simulink model "LKAS_AutoSave_20200911_1102"  (R2018b)
settings: Solver=FixedStepDiscrete  StartTime=0.0  StopTime=10.0  FixedStep=0.01  RelTol=1e-3
InitFcn:
  | tmpVer = ver('MATLAB');
  | tmpVer = str2num(tmpVer.Version);
  | % -------------------------------------------------------------------
  | %  MATLAB file generated by Simulink.saveVars on 21-Nov-2019 10:06:14
  | %  MATLAB version: 7.13.0.564 (R2011b)
  | % -------------------------------------------------------------------
  | 
  | 
  | SInt16 = Simulink.AliasType;
  | SInt16.Description = 'Num';
  | if (tmpVer > 7.11)
  | 	SInt16.DataScope = 'Auto';
  | end
  | SInt16.HeaderFile = 'Rte_Type.h';
  | SInt16.BaseType = 'int16';
  | 
  | SInt32 = Simulink.AliasType;
  | SInt32.Description = 'Num';
  | if (tmpVer > 7.11)
  | 	SInt32.DataScope = 'Auto';
  | end
  | SInt32.HeaderFile = 'Rte_Type.h';
  | SInt32.BaseType = 'int32';
  | 
  | SInt8 = Simulink.AliasType;
  | SInt8.Description = 'Num';
  | if (tmpVer > 7.11)
  | 	SInt8.DataScope = 'Auto';
  | end
  | SInt8.HeaderFile = 'Rte_Type.h';
  | SInt8.BaseType = 'int8';
  | 
  | T_A_m2_1024_1_u32 = Simulink.NumericType;
  | T_A_m2_1024_1_u32.Description = 'm2 (square meters  (m2))';
  | if (tmpVer > 7.11)
  | 	T_A_m2_1024_1_u32.DataScope = 'Auto';
  | end
  | T_A_m2_1024_1_u32.HeaderFile = 'Rte_Type.h';
  | T_A_m2_1024_1_u32.DataTypeMode = 'Fixed-point: slope and bias scaling';
  | T_A_m2_1024_1_u32.SignednessBool = false;
  | T_A_m2_1024_1_u32.WordLength = 32;
  | T_A_m2_1024_1_u32.FixedExponent = -10;
  | T_A_m2_1024_1_u32.SlopeAdjustmentFactor = 1;
  | T_A_m2_1024_1_u32.Bias = 0;
  | T_A_m2_1024_1_u32.DataTypeOverride = 'Inherit';
  | T_A_m2_1024_1_u32.IsAlias = true;
  | 
  | T_A_m2_65536_1_u16 = Simulink.NumericType;
  | T_A_m2_65536_1_u16.Description = 'm2 (square meters  (m2))';
  | if (tmpVer > 7.11)
  | 	T_A_m2_65536_1_u16.DataScope = 'Auto';
  | end
  | T_A_m2_65536_1_u16.HeaderFile = 'Rte_Type.h';
  | T_A_m2_65536_1_u16.DataTypeMode = 'Fixed-point: slope and bias scaling';
  | T_A_m2_65536_1_u16.SignednessBool = false;
  | T_A_m2_65536_1_u16.WordLength = 16;
  | T_A_m2_65536_1_u16.FixedExponent = -16;
  | T_A_m2_65536_1_u16.SlopeAdjustmentFactor = 1;
  | T_A_m2_65536_1_u16.Bias = 0;
  | T_A_m2_65536_1_u16.DataTypeOverride = 'Inherit';
  | ... (+4598 lines)
StopFcn:
  | clear  T_A_m2_1024_1_u32 T_A_m2_65536_1_u16 T_A_m2_Float32 T_A_mm2_10_1_u16 T_A_mm2_4_1_s16 T_A_mm2_Float32 T_Cnt_Num_10_1_u32 T_Cnt_Num_1_1_s16 T_Cnt_Num_1_1_s32 T_Cnt_Num_1_1_s8 T_Cnt_Num_1_1_u16 T_Cnt_Num_1_1_u32 T_Cnt_Num_1_1_u8 T_E_J_1_1_s32 T_E_J_Float32 T_E_kJ_128_1_s32 T_E_kJ_Float32 T_E_kwh_10_1_u16 T_E_kwh_Float32 T_Epl_kwhpkm_100_1_u16 T_Epl_kwhpkm_Float32 T_F_N_1_1_s16 T_F_N_Float32 T_I_A_1000_1_u16 T_I_A_1048576_1_s32 T_I_A_2048_1_s16 T_I_A_32_1_s16 T_I_A_Float32 T_I_mA_1_1_s16 T_I_mA_32768_128_s16 T_I_mA_Float32 T_J_kgpm2_128_1_u16 T_J_kgpm2_Float32 T_K_NA_1000_1_s16 T_K_NA_100_1_s16 T_K_NA_100_1_u16 T_K_NA_1024_1_s16 T_K_NA_1024_1_u16 T_K_NA_128_1_s16 T_K_NA_128_1_u16 T_K_NA_128_1_u8 T_K_NA_16777216_1_u32 T_K_NA_16_1_s16 T_K_NA_16_1_u16 T_K_NA_16_1_u8 T_K_NA_1_16_u16 T_K_NA_1_1_s16 T_K_NA_1_1_u16 T_K_NA_1_1_u8 T_K_NA_32768_1_s16 T_K_NA_32768_1_u16 T_K_NA_32_1_s8 T_K_NA_4096_1_u16 T_K_NA_4194304_1_s32 T_K_NA_4194304_1_u16 T_K_NA_65536_1_s32 T_K_NA_65536_1_u16 T_K_NA_8192_1_s16 T_K_NA_8_1_s16 T_K_NA_Float32 T_M_Nm_16_1_s16 T_M_Nm_1_1_s16 T_M_Nm_32768_1_s16 T_M_Nm_32_1_s16 T_M_Nm_4_1_s16 T_M_Nm_512_1_s16 T_M_Nm_Float32 T_P_W_1_4_s16 T_P_W_1_8_s16 T_P_W_Float32 T_P_kW_128_1_s16 T_P_kW_1_8_s16 T_P_kW_8_1_s32 T_P_kW_Float32 T_Pct_pct_1024_1_s32 T_Pct_pct_1024_1_u32 T_Pct_pct_10_1_s16 T_Pct_pct_10_1_u32 T_Pct_pct_128_100_s8 T_Pct_pct_1_1_s16 T_Pct_pct_1_4_u8 T_Pct_pct_255_100_u16 T_Pct_pct_255_100_u8 T_Pct_pct_256_1_s16 T_Pct_pct_256_1_u16 T_Pct_pct_65535_100_u16 T_Pct_pct_Float32 T_R_ohm_1024_1_s16 T_R_ohm_32_1_s16 T_R_ohm_Float32 T_TK_K_16_1_s16 T_TK_K_Float32 T_T_degC_10_400_1_u16 T_T_degC_16_1_s16 T_T_degC_1_40_1_u8 T_T_degC_2_80_1_u8 T_T_degC_Float32 T_U_V_1000_1_u16 T_U_V_10_1_u8 T_U_V_200_1_u8 T_U_V_32_1_s16 T_U_V_4096_1_s16 T_U_V_512_1_s16 T_U_V_65535_8_u16 T_U_V_8192_1_u16 T_U_V_Float32 T_U_mV_1_1_s16 T_U_mV_256_20_u16 T_U_mV_Float32 T_V_l_256_1_s16 T_V_l_4096_1_s16 T_V_l_64_1_s16 T_V_l_65535_100_u16 T_V_l_Float32 T_V_ml_128_1_s16 T_V_ml_1_1_s16 T_V_ml_32768_1_s16 T_V_ml_Float32 T_V_ul_32_1_u16 T_V_ul_Float32 T_Vpl_clpkm_512_1_u16 T_Vpl_clpkm_Float32 T_a_kphps_16_1_s16 T_a_kphps_Float32 T_a_mps2_128_1_s16 T_a_mps2_Float32 T_c_MJpkg_256_1_s16 T_c_MJpkg_Float32 T_c_kJpgpK_1024_1_s16 T_c_kJpgpK_Float32 T_c_kJpkgpK_128_1_u16 T_c_kJpkgpK_Float32 T_chrg_Ah_1_1_s16 T_chrg_Ah_1_1_u16 T_chrg_Ah_1_1_u8 T_chrg_Ah_256_1_u16 T_chrg_Ah_4194304_1_s32 T_chrg_Ah_512_1_u16 T_chrg_Ah_8_1_u16 T_chrg_Ah_Float32 T_cmp_NA_100_1_s16 T_cmp_NA_128_1_s16 T_cmp_NA_16_1_s16 T_cmp_NA_32768_1_u16 T_cmp_NA_Float32 T_d2n_rpmps2_4_1_s16 T_d2n_rpmps2_Float32 T_dPct_pctps_16_1_s16 T_dPct_pctps_256_1_s16 T_dPct_pctps_Float32 T_dT_degCps_128_1_s16 T_dT_degCps_Float32 T_dV_lph_1_1_s16 T_dV_lph_Float32 T_dV_lpm_128_1_s16 T_dV_lpm_32_1_s16 T_dV_lpm_Float32 T_dV_lps_1024_1_u16 T_dV_lps_4_1_u16 T_dV_lps_Float32 T_dV_mlps_1024_1_s16 T_dV_mlps_Float32 T_d_BitField16 T_dm_gps_128_1_s16 T_dm_gps_128_1_u16 T_dm_gps_256_1_u16 T_dm_gps_Float32 T_dm_mgps_1_1_s16 T_dm_mgps_Float32 T_dn_rpmps_1_1_s16 T_dn_rpmps_2_1_s16 T_dn_rpmps_Float32 T_dp_Paps_1_1_s16 T_dp_Paps_Float32 T_dp_kPaps_1_1_s16 T_dp_kPaps_8_1_s16 T_dp_kPaps_Float32 T_dphi_degps_128_1_s16 T_dphi_degps_8_1_s16 T_dphi_degps_Float32 T_dr_ps_256_1_s16 T_dr_ps_Float32 T_drho_mgplps_1_2_s16 T_drho_mgplps_Float32 T_e_NA_1_1_u8 T_f_Hz_1_1_u16 T_f_Hz_1_1_u32 T_f_Hz_64_1_u16 T_f_Hz_8_1_s16 T_f_Hz_Float32 T_g_BitField32 T_l_km_16_1_s16 T_l_km_1_1_u16 T_l_km_1_1_u32 T_l_km_Float32 T_l_m_1024_1_s16 T_l_m_16_1_s16 T_l_m_1_1_u32 T_l_m_Float32 T_l_mm_16_1_s16 T_l_mm_1_1_u16 T_l_mm_4096_1_s16 T_l_mm_4_1_u8 T_l_mm_64_1_s16 T_l_mm_Float32 T_m_g_1_1_s16 T_m_g_2048_1_s16 T_m_g_32_1_u16 T_m_g_Float32 T_m_kg_1024_1_s16 T_m_kg_1_1_s16 T_m_kg_1_1_u32 T_m_kg_Float32 T_m_mg_128_1_s16 T_m_mg_32_1_s16 T_m_mg_Float32 T_n_rpm_1_1_s16 T_n_rpm_1_25_u8 T_n_rpm_256_50_u16 T_n_rpm_2_25_u8 T_n_rpm_4_1_u16 T_n_rpm_Float32 T_p_MPa_64_1_s16 T_p_MPa_Float32 T_p_Pa_1_1_s16 T_p_Pa_Float32 T_p_kPa_1_10_u16 T_p_kPa_1_1_s16 T_p_kPa_1_1_u8 T_p_kPa_256_1_u16 T_p_kPa_32_1_u16 T_p_kPa_64_1_s16 T_p_kPa_Float32 T_phi_deg_100_1_s16 T_phi_deg_1024_1_s16 T_phi_deg_128_1_s16 T_phi_deg_1_1_u8 T_phi_deg_256_1_s16 T_phi_deg_2_1_s8 T_phi_deg_32_1_s16 T_phi_deg_512_6_s32 T_phi_deg_Float32 T_phi_rad_2048_1_s16 T_phi_rad_Float32 T_r_NA_1024_1_s16 T_r_NA_1024_1_u16 T_r_NA_16384_1_s16 T_r_NA_16_1_s16 T_r_NA_256_1_s8 T_r_NA_256_1_u16 T_r_NA_32768_1_u16 T_r_NA_32_1_u16 T_r_NA_4096_1_s16 T_r_NA_65535_2_u16 T_r_NA_8192_1_u16 T_r_NA_Float32 T_rho_gpl_8192_1_s16 T_rho_gpl_Float32 T_rho_kgpm3_16_1_s16 T_rho_kgpm3_Float32 T_rho_mgpl_1_1_s16 T_rho_mgpl_64_1_s16 T_rho_mgpl_Float32 T_t_hour_1_1_s16 T_t_hour_Float32 T_t_m_1_1_u16 T_t_m_Float32 T_t_ms_1_1_s16 T_t_ms_1_1_u16 T_t_ms_1_1_u32 T_t_ms_4096_1_s16 T_t_ms_64_1_s16 T_t_ms_Float32 T_t_s_1000_1_s16 T_t_s_100_1_s16 T_t_s_10_1_s16 T_t_s_10_1_u16 T_t_s_1_1_s16 T_t_s_1_1_u16 T_t_s_1_1_u32 T_t_s_Float32 T_t_us_10_1_u32 T_t_us_1_1_s16 T_t_us_1_1_u32 T_t_us_1_4_u16 T_t_us_Float32 T_v_kph_1_1_u8 T_v_kph_64_1_s16 T_v_kph_64_1_u16 T_v_kph_Float32 T_v_mps_256_1_s16 T_v_mps_Float32 T_w_radps_32_1_s16 T_w_radps_Float32 T_y_BitField8 T_y_BitFieldDiagProgress T_y_BitFieldDiagStatus T_y_NA_1_1_u8 SInt16 SInt32 SInt8 T_BOOLEAN UInt16 UInt32 UInt8 s16 s32 s8 u16 u32 u8
model workspace (MAT data in the model file):
  MCOS : class17 (value not decoded)
  MCOS : class17 (value not decoded)
  MCOS : class17 (value not decoded)
  MCOS : class17 (value not decoded)
  MCOS : class17 (value not decoded)
  MCOS : class17 (value not decoded)
  MCOS : class17 (value not decoded)
  MCOS : class17 (value not decoded)
  MCOS : class17 (value not decoded)
  MCOS : class17 (value not decoded)
  MCOS : class17 (value not decoded)
  MCOS : class17 (value not decoded)
  MCOS : class17 (value not decoded)
  MCOS : class17 (value not decoded)
  MCOS : class17 (value not decoded)
  MCOS : class17 (value not decoded)
  MCOS : class17 (value not decoded)
  MCOS : class17 (value not decoded)
  MCOS : class17 (value not decoded)
  MCOS : class17 (value not decoded)
  MCOS : class17 (value not decoded)
  MCOS : class17 (value not decoded)
  MCOS : class17 (value not decoded)
  MCOS : class17 (value not decoded)
  MCOS : class17 (value not decoded)
  MCOS : class17 (value not decoded)
  MCOS : class17 (value not decoded)
  MCOS : class17 (value not decoded)
  MCOS : class17 (value not decoded)
  MCOS : class17 (value not decoded)
  MCOS : class17 (value not decoded)
  MCOS : class17 (value not decoded)
  MCOS : class17 (value not decoded)
  MCOS : class17 (value not decoded)
  MCOS : class17 (value not decoded)
  MCOS : class17 (value not decoded)
  MCOS : class17 (value not decoded)
  MCOS : class17 (value not decoded)
  MCOS : class17 (value not decoded)
  MCOS : class17 (value not decoded)
  MCOS : class17 (value not decoded)
  MCOS : class17 (value not decoded)
  MCOS : class17 (value not decoded)
  MCOS : class17 (value not decoded)
  MCOS : class17 (value not decoded)
  MCOS : class17 (value not decoded)
  MCOS : class17 (value not decoded)
  MCOS : class17 (value not decoded)
  MCOS : class17 (value not decoded)
  MCOS : class17 (value not decoded)
  MCOS : class17 (value not decoded)
  MCOS : class17 (value not decoded)
  MCOS : class17 (value not decoded)
  MCOS : class17 (value not decoded)
  MCOS : class17 (value not decoded)
  MCOS : class17 (value not decoded)
  MCOS : class17 (value not decoded)
  MCOS : class17 (value not decoded)
  MCOS : class17 (value not decoded)
  MCOS : class17 (value not decoded)
  MCOS : class17 (value not decoded)
  MCOS : class17 (value not decoded)
  MCOS : class17 (value not decoded)
  MCOS : class17 (value not decoded)
  MCOS : class17 (value not decoded)
  MCOS : class17 (value not decoded)
  MCOS : class17 (value not decoded)
  MCOS : class17 (value not decoded)
  MCOS : class17 (value not decoded)
  MCOS : class17 (value not decoded)
  MCOS : class17 (value not decoded)
  MCOS : class17 (value not decoded)
  MCOS : class17 (value not decoded)
  MCOS : class17 (value not decoded)
  MCOS : class17 (value not decoded)
  MCOS : class17 (value not decoded)
  MCOS : class17 (value not decoded)
  MCOS : class17 (value not decoded)
  MCOS : class17 (value not decoded)
  MCOS : class17 (value not decoded)
  MCOS : class17 (value not decoded)
  MCOS : class17 (value not decoded)
  MCOS : class17 (value not decoded)
  MCOS : class17 (value not decoded)
  MCOS : class17 (value not decoded)
  MCOS : class17 (value not decoded)
  MCOS : class17 (value not decoded)
  MCOS : class17 (value not decoded)
  MCOS : class17 (value not decoded)
undefined symbols (not defined in the file): LKA_CarWidth, LKA_SampleTime, LKA_StrRatio_C, LKA_Veh2CamL_C, LKA_Veh2CamW_C, LKA_WhlBaseL_C, LL_CompSWA_C, LL_CrvtPrvwT_C, LL_DesDvt_C, LL_DvtComp_C, LL_DvtPrvwT_C, LL_DvtSpdDet_vDvtSpdMin_C, LL_HdAgExT_C, LL_HdAgPrvwT_C, LL_LAccMax_C, LL_LAccRMax_C, LL_LDW_EarliestWarnLine_C, LL_LDW_LatestWarnLine_C, LL_LDWS_SUPPRESS_HEADING, LL_LFClb_TFC_DiffCtlBalance, LL_LFClb_TFC_DiffCtrlMaxSWA, LL_LFClb_TFC_DiffCtrlRatio, LL_LFClb_TFC_facmGainLutGain1_C, LL_LFClb_TFC_facmGainLutGain2_C, LL_LFClb_TFC_facmIntegRatio, LL_LFClb_TFC_facmKlat_C, LL_LFClb_TFC_FfCtlRatio_C, LL_LFClb_TFC_phiIntegCtlMaxSWA_C, LL_LFClb_TFC_tiKlatPrvwT_C, LL_LFClb_TFC_vGainLutVehSpdLwr_C, LL_LFClb_TFC_vGainLutVehSpdUpr_C, LL_LKA_EarliestWarnLine_C, LL_LKA_LatestWarnLine_C, LL_LKAExPrcs_ExitC0Dvt, LL_LKAExPrcs_ExitC0Swt, LL_LKAExPrcs_tiExitTime1, LL_LKAExPrcs_tiExitTime2, LL_LKAExPrcs_tiExitTime3, LL_LKAS_OUT_OF_CONTROL_LAT_VEL, LL_LKAS_OUT_OF_CONTROL_TTLC, LL_LKASWASyn_M0, LL_LKASWASyn_M1, LL_LKASWASyn_M2, LL_LKASWASyn_M3K, LL_LKASWASyn_SWAaddMax, LL_LKASWASyn_T2, LL_LKASWASyn_tiTrqSwaRtTime, LL_LKASWASyn_tiTrqSwaTime, LL_LKASWASyn_TrqMax, LL_LKASWASyn_TrqSwaAddSwt, LL_LKASWASyn_TrqSwaRateDiff, LL_LSpdCompT_C, LL_lStpLngth_C, LL_MAX_DELAY_EPSSTAR_TIME, LL_MAX_DRIVER_TORQUE_DISABLE, LL_MAX_DRIVER_TORQUE_ENABLE, LL_MAX_LANE_WIDTH_DISABLE, LL_MAX_LANE_WIDTH_ENABLE, LL_MAX_LAT_ACC_DISABLE, LL_MAX_LAT_ACC_ENABLE ... (+29)
libraries: simulink x134, dspstat3 x3, simulink_extras x1
(part 11 of 19)

== system LKAS_AutoSave_20200911_1102/LKAS/LL/LLOn/LKA/LKA Exit Processing (LKAExPrcs)/Exit Time 3/Moving Standard Deviation2 ==
  In1 : Inport
  Delay{,1..48} (49 alike) : Delay  DelayLength=1
  Mux : Mux  Inputs=50
  Standard Deviation : dspstat3/Standard Deviation  run=off  directionMode=Entire input  dimension=2  reset_popup=None  roiEnable=off  roiType=Rectangles  roiPortion=Entire ROI  roiOutput=Individual statistics for each ROI  roiFlag=off
      settings: SourceProductName=DSP System Toolbox  SourceProductBaseCode=DS
  Out1 : Outport
  wires:
  In1/1 -> Mux/1, Delay/1
  Delay2/1 -> Mux/4, Delay3/1
  Delay1/1 -> Mux/3, Delay2/1
  Mux/1 -> Standard Deviation/1
  Delay/1 -> Mux/2, Delay1/1
  Standard Deviation/1 -> Out1/1
  Delay3/1 -> Mux/5, Delay4/1
  Delay4/1 -> Mux/6, Delay5/1
  Delay7/1 -> Mux/9, Delay8/1
  Delay6/1 -> Mux/8, Delay7/1
  Delay5/1 -> Mux/7, Delay6/1
  Delay8/1 -> Delay9/1, Mux/10
  Delay18/1 -> Delay28/1, Mux/20
  Delay15/1 -> Mux/17, Delay16/1
  Delay16/1 -> Mux/18, Delay17/1
  Delay17/1 -> Mux/19, Delay18/1
  Delay14/1 -> Mux/16, Delay15/1
  Delay13/1 -> Mux/15, Delay14/1
  Delay10/1 -> Mux/12, Delay11/1
  Delay11/1 -> Mux/13, Delay12/1
  Delay12/1 -> Mux/14, Delay13/1
  Delay9/1 -> Mux/11, Delay10/1
  Delay28/1 -> Mux/21, Delay19/1
  Delay21/1 -> Mux/24, Delay22/1
  Delay20/1 -> Mux/23, Delay21/1
  Delay19/1 -> Mux/22, Delay20/1
  Delay22/1 -> Mux/25, Delay23/1
  Delay23/1 -> Mux/26, Delay24/1
  Delay26/1 -> Mux/29, Delay27/1
  Delay25/1 -> Mux/28, Delay26/1
  Delay24/1 -> Mux/27, Delay25/1
  Delay27/1 -> Delay38/1, Mux/30
  Delay37/1 -> Delay48/1, Mux/40
  Delay34/1 -> Mux/37, Delay35/1
  Delay35/1 -> Mux/38, Delay36/1
  Delay36/1 -> Mux/39, Delay37/1
  Delay33/1 -> Mux/36, Delay34/1
  Delay32/1 -> Mux/35, Delay33/1
  Delay29/1 -> Mux/32, Delay30/1
  Delay30/1 -> Mux/33, Delay31/1
  Delay31/1 -> Mux/34, Delay32/1
  Delay38/1 -> Mux/31, Delay29/1
  Delay48/1 -> Mux/41, Delay39/1
  Delay41/1 -> Mux/44, Delay42/1
  Delay40/1 -> Mux/43, Delay41/1
  Delay39/1 -> Mux/42, Delay40/1
  Delay42/1 -> Mux/45, Delay43/1
  Delay43/1 -> Mux/46, Delay44/1
  Delay46/1 -> Mux/49, Delay47/1
  Delay45/1 -> Mux/48, Delay46/1
  Delay44/1 -> Mux/47, Delay45/1
  Delay47/1 -> Mux/50

== system LKAS_AutoSave_20200911_1102/LKAS/LL/LLOn/LKA/LKA Exit Processing (LKAExPrcs)/Exit Time 3/Sum Condition ==
  In : Inport
  In1 : Inport  Port=2
  Enable : EnablePort  StatesWhenEnabling=reset
  Add1 : Sum  OutDataTypeStr=single
  Data Type Conversion : DataTypeConversion  OutDataTypeStr=uint16
  Memory : Memory  InheritSampleTime=on
  Relational Operator : RelationalOperator  OutDataTypeStr=boolean  RndMeth=Nearest
  Saturation : Saturate  UpperLimit=100000  LowerLimit=0
  Out : Outport  OutputWhenDisabled=reset  InitialOutput=0
  wires:
  Saturation/1 -> Memory/1, Relational Operator/1
  Relational Operator/1 -> Data Type Conversion/1
  Memory/1 -> Add1/2
  Add1/1 -> Saturation/1
  In/1 -> Add1/1
  In1/1 -> Relational Operator/2
  Data Type Conversion/1 -> Out/1

== system LKAS_AutoSave_20200911_1102/LKAS/LL/LLOn/LKA/LKA Exit Processing (LKAExPrcs)/Exit Time 3/Sum Condition1 ==
  In : Inport
  In1 : Inport  Port=2
  Enable : EnablePort  StatesWhenEnabling=reset
  Add1 : Sum  OutDataTypeStr=single
  Data Type Conversion : DataTypeConversion  OutDataTypeStr=uint16
  Memory : Memory  InheritSampleTime=on
  Relational Operator : RelationalOperator  OutDataTypeStr=boolean  RndMeth=Nearest
  Saturation : Saturate  UpperLimit=100000  LowerLimit=0
  Out : Outport  OutputWhenDisabled=reset  InitialOutput=0
  wires:
  Data Type Conversion/1 -> Out/1
  In1/1 -> Relational Operator/2
  In/1 -> Add1/1
  Add1/1 -> Saturation/1
  Memory/1 -> Add1/2
  Relational Operator/1 -> Data Type Conversion/1
  Saturation/1 -> Relational Operator/1, Memory/1

== system LKAS_AutoSave_20200911_1102/LKAS/LL/LLOn/LKA/LKA Motion Planning (LKAMP) /LKA Motion Planning Calculation (LKAMPCal)/Time Division (TDiv) ==
  TDiv_bsTDivInfoOut : Inport
  Add : Sum  OutDataTypeStr=uint16
  Constant : Constant  OutDataTypeStr=uint16  SampleTime=-1
  Constant19 : Constant  OutDataTypeStr=uint16  SampleTime=-1
  If : If  NumInputs=2  IfExpression=u1==u2
  Memory : Memory  InheritSampleTime=on
  Merge : Merge
  Saturation1 : Saturate  UpperLimit=100  LowerLimit=0  OutDataTypeStr=uint16
  if action 1 : Subsystem  TreatAsAtomicUnit=on
  if action 2 : Subsystem  TreatAsAtomicUnit=on
  Out1 : Outport
  wires:
  TDiv_bsTDivInfoOut/1 -> if action 1/1(In1)
  if action 1/1(Out1) -> Merge/2
  Merge/1 -> Out1/1
  if action 2/1(Out1) -> Merge/1
  If/1 -> if action 2/Action
  If/2 -> if action 1/Action
  Memory/1 -> Add/2
  Constant/1 -> Add/1
  Constant19/1 -> If/2
  Add/1 -> Memory/1, Saturation1/1
  Saturation1/1 -> If/1

== system LKAS_AutoSave_20200911_1102/LKAS/LL/LLOn/LKA/LKA Motion Planning (LKAMP) /LKA Motion Planning Calculation (LKAMPCal)/Time Division (TDiv)1 ==
  TDiv_bsTDivInfoOut1 : Inport
  Add : Sum  OutDataTypeStr=uint16
  Constant : Constant  OutDataTypeStr=uint16  SampleTime=-1
  Constant19 : Constant  OutDataTypeStr=uint16  SampleTime=-1
  If : If  NumInputs=2  IfExpression=u1==u2
  Memory : Memory  InheritSampleTime=on
  Merge1 : Merge
  Saturation1 : Saturate  UpperLimit=100  LowerLimit=0  OutDataTypeStr=uint16
  if action 3 : Subsystem  TreatAsAtomicUnit=on
  if action 4 : Subsystem  TreatAsAtomicUnit=on
  Out2 : Outport
  wires:
  Merge1/1 -> Out2/1
  TDiv_bsTDivInfoOut1/1 -> if action 3/1(In1)
  if action 4/1(Out1) -> Merge1/1
  if action 3/1(Out1) -> Merge1/2
  If/2 -> if action 3/Action
  Saturation1/1 -> If/1
  Add/1 -> Saturation1/1, Memory/1
  Constant19/1 -> If/2
  Constant/1 -> Add/1
  Memory/1 -> Add/2
  If/1 -> if action 4/Action

== system LKAS_AutoSave_20200911_1102/LKAS/LL/LLOn/LKA/LKA Motion Planning (LKAMP) /LKA Motion Planning Calculation (LKAMPCal)/Time Division (TDiv)2 ==
  TDiv_bsTDivInfoOut1 : Inport
  Add : Sum  OutDataTypeStr=uint16
  Constant : Constant  OutDataTypeStr=uint16  SampleTime=-1
  Constant19 : Constant  OutDataTypeStr=uint16  SampleTime=-1
  If : If  NumInputs=2  IfExpression=u1==u2
  Memory : Memory  InheritSampleTime=on
  Merge1 : Merge
  Saturation1 : Saturate  UpperLimit=100  LowerLimit=0  OutDataTypeStr=uint16
  if action 3 : Subsystem  TreatAsAtomicUnit=on
  if action 4 : Subsystem  TreatAsAtomicUnit=on
  Out2 : Outport
  wires:
  If/1 -> if action 4/Action
  Memory/1 -> Add/2
  Constant/1 -> Add/1
  Constant19/1 -> If/2
  Add/1 -> Memory/1, Saturation1/1
  Saturation1/1 -> If/1
  If/2 -> if action 3/Action
  if action 3/1(Out1) -> Merge1/2
  if action 4/1(Out1) -> Merge1/1
  TDiv_bsTDivInfoOut1/1 -> if action 3/1(In1)
  Merge1/1 -> Out2/1

== system LKAS_AutoSave_20200911_1102/LKAS/LL/LLOn/LKA/LKA Motion Planning (LKAMP) /LKA Motion Planning Calculation (LKAMPCal)/Time Division (TDiv)3 ==
  TDiv_bsTDivInfoOut1 : Inport
  Add : Sum  OutDataTypeStr=uint16
  Constant : Constant  OutDataTypeStr=uint16  SampleTime=-1
  Constant19 : Constant  OutDataTypeStr=uint16  SampleTime=-1
  If : If  NumInputs=2  IfExpression=u1==u2
  Memory : Memory  InheritSampleTime=on
  Merge1 : Merge
  Saturation1 : Saturate  UpperLimit=100  LowerLimit=0  OutDataTypeStr=uint16
  if action 3 : Subsystem  TreatAsAtomicUnit=on
  if action 4 : Subsystem  TreatAsAtomicUnit=on
  Out2 : Outport
  wires:
  Merge1/1 -> Out2/1
  TDiv_bsTDivInfoOut1/1 -> if action 3/1(In1)
  if action 4/1(Out1) -> Merge1/1
  if action 3/1(Out1) -> Merge1/2
  If/2 -> if action 3/Action
  Saturation1/1 -> If/1
  Add/1 -> Saturation1/1, Memory/1
  Constant19/1 -> If/2
  Constant/1 -> Add/1
  Memory/1 -> Add/2
  If/1 -> if action 4/Action

== system LKAS_AutoSave_20200911_1102/LKAS/LL/LLOn/LKA/LKA Motion Planning (LKAMP) /LKA Motion Planning Calculation (LKAMPCal)/Time Division (TDiv)4 ==
  TDiv_bsTDivInfoOut1 : Inport
  Add : Sum  OutDataTypeStr=uint16
  Constant : Constant  OutDataTypeStr=uint16  SampleTime=-1
  Constant19 : Constant  OutDataTypeStr=uint16  SampleTime=-1
  If : If  NumInputs=2  IfExpression=u1==u2
  Memory : Memory  InheritSampleTime=on
  Merge1 : Merge
  Saturation1 : Saturate  UpperLimit=100  LowerLimit=0  OutDataTypeStr=uint16
  if action 3 : Subsystem  TreatAsAtomicUnit=on
  if action 4 : Subsystem  TreatAsAtomicUnit=on
  Out2 : Outport
  wires:
  If/1 -> if action 4/Action
  Memory/1 -> Add/2
  Constant/1 -> Add/1
  Constant19/1 -> If/2
  Add/1 -> Memory/1, Saturation1/1
  Saturation1/1 -> If/1
  If/2 -> if action 3/Action
  if action 3/1(Out1) -> Merge1/2
  if action 4/1(Out1) -> Merge1/1
  TDiv_bsTDivInfoOut1/1 -> if action 3/1(In1)
  Merge1/1 -> Out2/1

== system LKAS_AutoSave_20200911_1102/LKAS/LL/LLOn/LKA/LKA Motion Planning (LKAMP) /Motion Planning Input Processing (MPInP)/Lane Information Selection (LaneInfoSel) ==
  LaneInfoSel_stLKAActvFlg : Inport
  LaneInfoSel_facmLftLane : Inport  Port=2
  LaneInfoSel_facmRgtLane : Inport  Port=3
  If : If  IfExpression=u1==1  ElseIfExpressions=u1==2
  If Action Subsystem1 : Subsystem  TreatAsAtomicUnit=on
  If Action Subsystem2 : Subsystem  TreatAsAtomicUnit=on
  If Action Subsystem3 : Subsystem  TreatAsAtomicUnit=on
  Merge : Merge  Inputs=3
  LaneInfoSel_facmActvLane : Outport
  wires:
  LaneInfoSel_facmRgtLane/1 -> If Action Subsystem1/1(In1)
  LaneInfoSel_facmLftLane/1 -> If Action Subsystem2/1(In1)
  LaneInfoSel_stLKAActvFlg/1 -> If/1
  If/1 -> If Action Subsystem2/Action
  If Action Subsystem2/1(Out1) -> Merge/1
  Merge/1 -> LaneInfoSel_facmActvLane/1
  If/2 -> If Action Subsystem1/Action
  If Action Subsystem1/1(Out1) -> Merge/2
  If Action Subsystem3/1(Out1) -> Merge/3
  If/3 -> If Action Subsystem3/Action

== system LKAS_AutoSave_20200911_1102/LKAS/LL/LLOn/LKA/LKA Motion Planning (LKAMP) /Motion Planning Input Processing (MPInP)/Signal Latching2 ==
  In : Inport
  Add : Sum  OutDataTypeStr=uint16
  Constant : Constant  OutDataTypeStr=uint16  SampleTime=-1
  Constant2 : Constant  Value=LatchTime  OutDataTypeStr=uint16  SampleTime=-1
  If : If  NumInputs=2  IfExpression=u1==u2  ShowElse=off
  Memory : Memory  InheritSampleTime=on
  Saturation1 : Saturate  UpperLimit=10000  LowerLimit=0  OutDataTypeStr=uint16
  "if action " : Subsystem  TreatAsAtomicUnit=on
  Out : Outport
  wires:
  Constant2/1 -> If/2
  In/1 -> "if action "/1(In)
  "if action "/1(Out) -> Out/1
  If/1 -> "if action "/Action
  Constant/1 -> Add/1
  Add/1 -> Saturation1/1
  Memory/1 -> Add/2
  Saturation1/1 -> Memory/1, If/1

== system LKAS_AutoSave_20200911_1102/LKAS/LL/LLOn/LKA/LKA Motion Planning (LKAMP) /Motion Planning Input Processing (MPInP)/Signal Latching3 ==
  In : Inport
  Add : Sum  OutDataTypeStr=uint16
  Constant : Constant  OutDataTypeStr=uint16  SampleTime=-1
  Constant2 : Constant  Value=LatchTime  OutDataTypeStr=uint16  SampleTime=-1
  If : If  NumInputs=2  IfExpression=u1==u2  ShowElse=off
  Memory : Memory  InheritSampleTime=on
  Saturation1 : Saturate  UpperLimit=10000  LowerLimit=0  OutDataTypeStr=uint16
  "if action " : Subsystem  TreatAsAtomicUnit=on
  Out : Outport
  wires:
  Saturation1/1 -> If/1, Memory/1
  Memory/1 -> Add/2
  Add/1 -> Saturation1/1
  Constant/1 -> Add/1
  If/1 -> "if action "/Action
  "if action "/1(Out) -> Out/1
  In/1 -> "if action "/1(In)
  Constant2/1 -> If/2

== system LKAS_AutoSave_20200911_1102/LKAS/LL/LLOn/LKA/LKA Motion Planning (LKAMP) /Motion Planning Input Processing (MPInP)/Signal Latching4 ==
  In : Inport
  Add : Sum  OutDataTypeStr=uint16
  Constant : Constant  OutDataTypeStr=uint16  SampleTime=-1
  Constant2 : Constant  Value=LatchTime  OutDataTypeStr=uint16  SampleTime=-1
  If : If  NumInputs=2  IfExpression=u1==u2  ShowElse=off
  Memory : Memory  InheritSampleTime=on
  Saturation1 : Saturate  UpperLimit=10000  LowerLimit=0  OutDataTypeStr=uint16
  "if action " : Subsystem  TreatAsAtomicUnit=on
  Out : Outport
  wires:
  Constant2/1 -> If/2
  In/1 -> "if action "/1(In)
  "if action "/1(Out) -> Out/1
  If/1 -> "if action "/Action
  Constant/1 -> Add/1
  Add/1 -> Saturation1/1
  Memory/1 -> Add/2
  Saturation1/1 -> Memory/1, If/1

== system LKAS_AutoSave_20200911_1102/LKAS/LL/LLOn/LKA/LKA Motion Planning (LKAMP) /Motion Planning Input Processing (MPInP)/Signal Latching5 ==
  In : Inport
  Add : Sum  OutDataTypeStr=uint16
  Constant : Constant  OutDataTypeStr=uint16  SampleTime=-1
  Constant2 : Constant  Value=LatchTime  OutDataTypeStr=uint16  SampleTime=-1
  If : If  NumInputs=2  IfExpression=u1==u2  ShowElse=off
  Memory : Memory  InheritSampleTime=on
  Saturation1 : Saturate  UpperLimit=10000  LowerLimit=0  OutDataTypeStr=uint16
  "if action " : Subsystem  TreatAsAtomicUnit=on
  Out : Outport
  wires:
  Constant2/1 -> If/2
  In/1 -> "if action "/1(In)
  "if action "/1(Out) -> Out/1
  If/1 -> "if action "/Action
  Constant/1 -> Add/1
  Add/1 -> Saturation1/1
  Memory/1 -> Add/2
  Saturation1/1 -> Memory/1, If/1

== system LKAS_AutoSave_20200911_1102/LKAS/LL/LLOn/LKA/LKA Motion Planning (LKAMP) /Motion Planning Input Processing (MPInP)/Signal Latching6 ==
  In : Inport
  Add : Sum  OutDataTypeStr=uint16
  Constant : Constant  OutDataTypeStr=uint16  SampleTime=-1
  Constant2 : Constant  Value=LatchTime  OutDataTypeStr=uint16  SampleTime=-1
  If : If  NumInputs=2  IfExpression=u1==u2  ShowElse=off
  Memory : Memory  InheritSampleTime=on
  Saturation1 : Saturate  UpperLimit=10000  LowerLimit=0  OutDataTypeStr=uint16
  "if action " : Subsystem  TreatAsAtomicUnit=on
  Out : Outport
  wires:
  Constant2/1 -> If/2
  In/1 -> "if action "/1(In)
  "if action "/1(Out) -> Out/1
  If/1 -> "if action "/Action
  Constant/1 -> Add/1
  Add/1 -> Saturation1/1
  Memory/1 -> Add/2
  Saturation1/1 -> Memory/1, If/1

== system LKAS_AutoSave_20200911_1102/LKAS/LL/LLOn/LKA/LKA Motion Planning (LKAMP) /Motion Planning Input Processing (MPInP)/Signal Latching7 ==
  In : Inport
  Add : Sum  OutDataTypeStr=uint16
  Constant : Constant  OutDataTypeStr=uint16  SampleTime=-1
  Constant2 : Constant  Value=LatchTime  OutDataTypeStr=uint16  SampleTime=-1
  If : If  NumInputs=2  IfExpression=u1==u2  ShowElse=off
  Memory : Memory  InheritSampleTime=on
  Saturation1 : Saturate  UpperLimit=10000  LowerLimit=0  OutDataTypeStr=uint16
  "if action " : Subsystem  TreatAsAtomicUnit=on
  Out : Outport
  wires:
  Saturation1/1 -> If/1, Memory/1
  Memory/1 -> Add/2
  Add/1 -> Saturation1/1
  Constant/1 -> Add/1
  If/1 -> "if action "/Action
  "if action "/1(Out) -> Out/1
  In/1 -> "if action "/1(In)
  Constant2/1 -> If/2

== system LKAS_AutoSave_20200911_1102/LKAS/LL/LLOn/LKA/LKA Motion Planning (LKAMP) /Motion Planning Input Processing (MPInP)/Subsystem ==
  In1 : Inport
  If : If  IfExpression=u1==1  ElseIfExpressions=u1==2
  If Action Subsystem1 : Subsystem  TreatAsAtomicUnit=on
  If Action Subsystem2 : Subsystem  TreatAsAtomicUnit=on
  If Action Subsystem3 : Subsystem  TreatAsAtomicUnit=on
  Merge : Merge  Inputs=3
  Out6 : Outport
  wires:
  If/3 -> If Action Subsystem3/Action
  If Action Subsystem3/1(Out1) -> Merge/3
  If Action Subsystem1/1(Out1) -> Merge/2
  If/2 -> If Action Subsystem1/Action
  Merge/1 -> Out6/1
  If Action Subsystem2/1(Out1) -> Merge/1
  If/1 -> If Action Subsystem2/Action
  In1/1 -> If/1

== system LKAS_AutoSave_20200911_1102/LKAS/LL/LLOn/LKA/LKA Motion Planning (LKAMP) /Switching Condition (SwtCon)/Ending Heading Angle Determination (EndHdAgDet) ==
  EndHdAgDet_stLKAActvFlg : Inport
  EndHdAgDet_vVehSpd : Inport  Port=2
  EndHdAgDet_crPrvwCrvt : Inport  Port=3
  EndHdAgDet_lLaneWidth_C : Inport  Port=4
  EndHdAgDet_lCarWidth_C : Inport  Port=5
  EndHdAgDet_tiHdAgExTime_C : Inport  Port=6
  EndHdAgDet_tiLSpdCompT_C : Inport  Port=7
  Add : Sum  Inputs=+-  OutDataTypeStr=single
  Add1 : Sum  OutDataTypeStr=single
  Divide : Product  Inputs=/*  OutDataTypeStr=single
  Divide1 : Product  Inputs=*/  OutDataTypeStr=single
  Lateral Speed Compensation (LSpdComp) : Subsystem
  kph To mps : Gain  Gain=1/3.6  OutDataTypeStr=single
  EndHdAgDet_phiHdAgMax : Outport
  wires:
  EndHdAgDet_tiLSpdCompT_C/1 -> Lateral Speed Compensation (LSpdComp)/4(LSpdComp_tiLSpdCompT_C)
  EndHdAgDet_crPrvwCrvt/1 -> Lateral Speed Compensation (LSpdComp)/3(LSpdComp_crPrvwCrvt)
  Add1/1 -> EndHdAgDet_phiHdAgMax/1
  Divide1/1 -> Add1/1
  Lateral Speed Compensation (LSpdComp)/1(LSpdComp_phiLSpdComp) -> Add1/2
  Add/1 -> Divide/2
  EndHdAgDet_stLKAActvFlg/1 -> Lateral Speed Compensation (LSpdComp)/2(LSpdComp_stLKAFlg)
  EndHdAgDet_vVehSpd/1 -> kph To mps/1
  EndHdAgDet_tiHdAgExTime_C/1 -> Divide/1
  kph To mps/1 -> Divide1/2, Lateral Speed Compensation (LSpdComp)/1(LSpdComp_vVehSpd)
  EndHdAgDet_lCarWidth_C/1 -> Add/2
  EndHdAgDet_lLaneWidth_C/1 -> Add/1
  Divide/1 -> Divide1/1

== system LKAS_AutoSave_20200911_1102/LKAS/LL/LLOn/LKA/LKA Motion Planning (LKAMP) /Switching Condition (SwtCon)/If Action Subsystem ==
  In1 : Inport
  Action Port : ActionPort  InitializeStates=reset  ActionType=then
  Gain2 : Gain  Gain=-1  OutDataTypeStr=Inherit: Same as input
  Out1 : Outport
  wires:
  In1/1 -> Gain2/1
  Gain2/1 -> Out1/1  "HdAgMax"

== system LKAS_AutoSave_20200911_1102/LKAS/LL/LLOn/LKA/LKA Motion Planning (LKAMP) /Switching Condition (SwtCon)/If Action Subsystem1 ==
  In1 : Inport
  Action Port : ActionPort  InitializeStates=reset  ActionType=elseif
  Cast To Single1 : DataTypeConversion  LockScale=on
  Out1 : Outport
  wires:
  In1/1 -> Cast To Single1/1
  Cast To Single1/1 -> Out1/1  "HdAgMax"

== system LKAS_AutoSave_20200911_1102/LKAS/LL/LLOn/LKA/LKA Motion Planning (LKAMP) /Switching Condition (SwtCon)/If Action Subsystem2 ==
  Action Port : ActionPort  InitializeStates=reset  ActionType=else
  Constant2 : Constant  Value=0  OutDataTypeStr=single  SampleTime=-1
  Out1 : Outport
  wires:
  Constant2/1 -> Out1/1  "HdAgMax"

== system LKAS_AutoSave_20200911_1102/LKAS/LL/LLOn/LKA/LKA Motion Planning (LKAMP) /Switching Condition (SwtCon)/Signal Latching ==
  In : Inport
  Add : Sum  OutDataTypeStr=uint16
  Constant : Constant  OutDataTypeStr=uint16  SampleTime=-1
  Constant2 : Constant  Value=LatchTime  OutDataTypeStr=uint16  SampleTime=-1
  If : If  NumInputs=2  IfExpression=u1==u2  ShowElse=off
  Memory : Memory  InheritSampleTime=on
  Saturation1 : Saturate  UpperLimit=10000  LowerLimit=0  OutDataTypeStr=uint16
  "if action " : Subsystem  TreatAsAtomicUnit=on
  Out : Outport
  wires:
  Constant2/1 -> If/2
  In/1 -> "if action "/1(In)
  "if action "/1(Out) -> Out/1
  If/1 -> "if action "/Action
  Constant/1 -> Add/1
  Add/1 -> Memory/1, Saturation1/1
  Memory/1 -> Add/2
  Saturation1/1 -> If/1

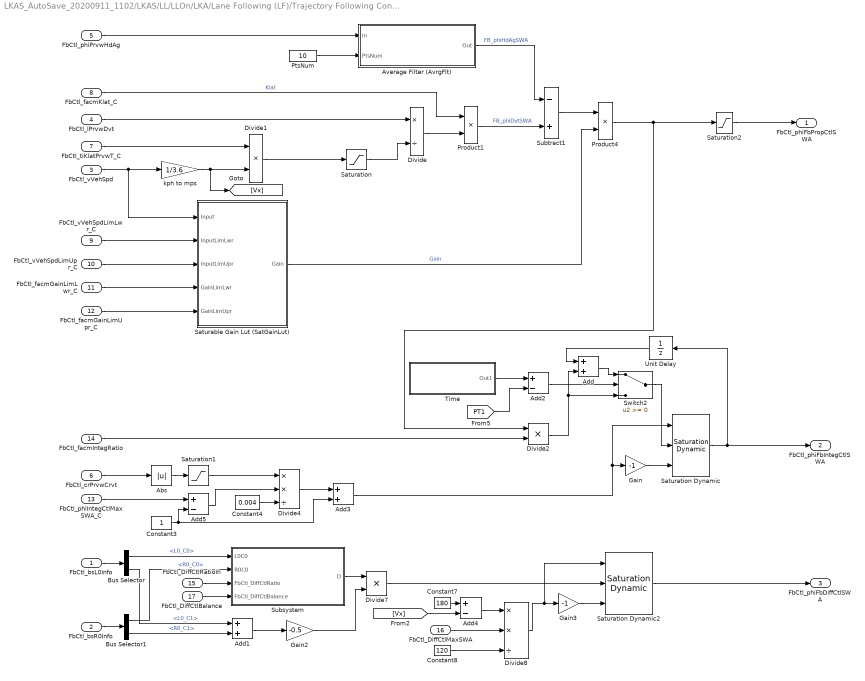
== system LKAS_AutoSave_20200911_1102/LKAS/LL/LLOn/LKA/Lane Following (LF)/Trajectory Following Control (TFC)/Feedback Control (FbCtl) ==
  FbCtl_bsL0Info : Inport
  FbCtl_bsR0Info : Inport  Port=2
  FbCtl_vVehSpd : Inport  Port=3
  FbCtl_lPrvwDvt : Inport  Port=4
  FbCtl_phiPrvwHdAg : Inport  Port=5
  FbCtl_crPrvwCrvt : Inport  Port=6
  FbCtl_tiKlatPrvwT_C : Inport  Port=7
  FbCtl_facmKlat_C : Inport  Port=8
  FbCtl_vVehSpdLimLwr_C : Inport  Port=9
  FbCtl_vVehSpdLimUpr_C : Inport  Port=10
  FbCtl_facmGainLimLwr_C : Inport  Port=11
  FbCtl_facmGainLimUpr_C : Inport  Port=12
  FbCtl_phiIntegCtlMaxSWA_C : Inport  Port=13
  FbCtl_facmIntegRatio : Inport  Port=14
  FbCtl_DiffCtlRatioIn : Inport  Port=15
  FbCtl_DiffCtlMaxSWA : Inport  Port=16
  FbCtl_DiffCtlBalance : Inport  Port=17
  Abs : Abs
  Add : Sum
  Add1 : Sum
  Add2 : Sum  Inputs=+-
  Add3 : Sum
  Add4 : Sum  Inputs=+-
  Add5 : Sum  Inputs=+-
  Average Filter (AvrgFlt) : Subsystem
      mask Display:
      | port_label('input', 1, 'In');
      | port_label('input', 2, 'PtsNum');
      | port_label('output', 1, 'Out');
      | color('blue');
      | text(0.98,0.9,'VCDC Block','horizontalAlignment','right');
      | color('black');
      | text(0.5,0.55,'Average Filter','horizontalAlignment','center');
      | text(0.5,0.4,'(AvrgFlt)','horizontalAlignment','center');
  Bus Selector : BusSelector  OutputSignals=L0_C0,L0_C1
  Bus Selector1 : BusSelector  OutputSignals=R0_C0,R0_C1
  Constant3 : Constant  OutDataTypeStr=single
  Constant4 : Constant  Value=0.004  OutDataTypeStr=single
  Constant7 : Constant  Value=180  OutDataTypeStr=single
  Constant8 : Constant  Value=120  OutDataTypeStr=single
  Divide : Product  Inputs=*/
  Divide1 : Product  Inputs=**
  Divide2 : Product  Inputs=**
  Divide4 : Product  Inputs=**/
  Divide7 : Product  Inputs=**
  Divide8 : Product  Inputs=**/
  Gain : Gain  Gain=-1  OutDataTypeStr=single
  Gain2 : Gain  Gain=-0.5
  Gain3 : Gain  Gain=-1  OutDataTypeStr=single
  Product1 : Product  OutDataTypeStr=single  RndMeth=Zero
  Product4 : Product  OutDataTypeStr=single  RndMeth=Zero
  PtsNum : Constant  Value=10  OutDataTypeStr=single
  Saturable Gain Lut (SatGainLut) : MATLAB Function  TreatAsAtomicUnit=on
  Saturation : Saturate  UpperLimit=40  LowerLimit=5
  Saturation Dynamic : simulink/Discontinuities/Saturation Dynamic  OutMin=[]  OutMax=[]  OutDataTypeStr=Inherit: Same as second input  OutDataType=fixdt(1, 16)  OutScaling=2^-10  DoSatur=off
  Saturation Dynamic2 : simulink/Discontinuities/Saturation Dynamic  OutMin=[]  OutMax=[]  OutDataTypeStr=Inherit: Same as second input  OutDataType=fixdt(1, 16)  OutScaling=2^-10  DoSatur=off
  Saturation1 : Saturate  UpperLimit=0.004  LowerLimit=0.00001
  Saturation2 : Saturate  UpperLimit=360  LowerLimit=-360  OutDataTypeStr=single
  Subsystem : Subsystem
  Subtract1 : Sum  Inputs=-+
  Switch2 : Switch
  Time : Subsystem
      mask Display:
      | port_label('output', 1, 'TTime');
      | color('blue');
      | text(0.98,0.9,'VCDC Block','horizontalAlignment','right');
      | color('black');
      | text(0.5,0.55,'Tick Time','horizontalAlignment','center');
      | text(0.5,0.4,'(TTime)','horizontalAlignment','center');
  Unit Delay : UnitDelay  SampleTime=-1
  kph to mps : Gain  Gain=1/3.6  OutDataTypeStr=single
  FbCtl_phiFbPropCtlSWA : Outport
  FbCtl_phiFbIntegCtlSWA : Outport  Port=2
  FbCtl_phiFbDiffCtlSWA : Outport  Port=3
  wires:
  Gain2/1 -> Divide7/2
  Bus Selector1/1 -> Subsystem/2(R0C0)  "<R0_C0>"
  Bus Selector/1 -> Subsystem/1(L0C0)  "<L0_C0>"
  FbCtl_bsR0Info/1 -> Bus Selector1/1
  FbCtl_bsL0Info/1 -> Bus Selector/1
  PtsNum/1 -> Average Filter (AvrgFlt)/2(PtsNum)
  FbCtl_facmKlat_C/1 -> Product1/1  "Klat"
  Product1/1 -> Subtract1/2  "FB_phiDvtSWA"
  Average Filter (AvrgFlt)/1(Out) -> Subtract1/1  "FB_phiHdAgSWA"
  Saturable Gain Lut (SatGainLut)/1(Gain) -> Product4/2  "Gain"
  Saturation2/1 -> FbCtl_phiFbPropCtlSWA/1
  Saturation/1 -> Divide/2
  Divide1/1 -> Saturation/1
  FbCtl_tiKlatPrvwT_C/1 -> Divide1/1
  FbCtl_lPrvwDvt/1 -> Divide/1
  Divide/1 -> Product1/2
  FbCtl_phiPrvwHdAg/1 -> Average Filter (AvrgFlt)/1(In)
  Product4/1 -> Divide2/1, Saturation2/1
  kph to mps/1 -> Divide1/2, [Vx]
  FbCtl_vVehSpdLimLwr_C/1 -> Saturable Gain Lut (SatGainLut)/2(InputLimLwr)
  FbCtl_vVehSpdLimUpr_C/1 -> Saturable Gain Lut (SatGainLut)/3(InputLimUpr)
  FbCtl_facmGainLimLwr_C/1 -> Saturable Gain Lut (SatGainLut)/4(GainLimLwr)
  FbCtl_facmGainLimUpr_C/1 -> Saturable Gain Lut (SatGainLut)/5(GainLimUpr)
  FbCtl_facmIntegRatio/1 -> Divide2/2
  Divide2/1 -> Add/2, Switch2/3
  Subtract1/1 -> Product4/1
  Add3/1 -> Saturation Dynamic/1, Gain/1
  FbCtl_phiIntegCtlMaxSWA_C/1 -> Add5/1
  FbCtl_vVehSpd/1 -> kph to mps/1, Saturable Gain Lut (SatGainLut)/1(Input)
  Unit Delay/1 -> Add/1
  Gain/1 -> Saturation Dynamic/3
  Saturation Dynamic/1 -> FbCtl_phiFbIntegCtlSWA/1, Unit Delay/1
  Divide7/1 -> Saturation Dynamic2/2
  Gain3/1 -> Saturation Dynamic2/3
  Divide8/1 -> Gain3/1, Saturation Dynamic2/1
  FbCtl_DiffCtlMaxSWA/1 -> Divide8/2
  Constant7/1 -> Add4/1
  Add4/1 -> Divide8/1
  Constant8/1 -> Divide8/3
  [Vx] -> Add4/2
  Bus Selector/2 -> Add1/1  "<L0_C1>"
  Add1/1 -> Gain2/1
  Bus Selector1/2 -> Add1/2  "<R0_C1>"
  Subsystem/1(D) -> Divide7/1
  FbCtl_DiffCtlRatioIn/1 -> Subsystem/3(FbCtl_DiffCtlRatio)
  Saturation Dynamic2/1 -> FbCtl_phiFbDiffCtlSWA/1
  Time/1(Out1) -> Add2/1
  [PT1] -> Add2/2
  Add2/1 -> Switch2/2
  Switch2/1 -> Saturation Dynamic/2
  Add/1 -> Switch2/1
  FbCtl_crPrvwCrvt/1 -> Abs/1
  Abs/1 -> Saturation1/1
  Constant3/1 -> Add5/2, Add3/2
  Saturation1/1 -> Divide4/1
  Divide4/1 -> Add3/1
  Constant4/1 -> Divide4/3
  Add5/1 -> Divide4/2
  FbCtl_DiffCtlBalance/1 -> Subsystem/4(FbCtl_DiffCtlBalance)

== system LKAS_AutoSave_20200911_1102/LKAS/LL/LLOn/LKA/Lane Following (LF)/Trajectory Following Control (TFC)/Feedforward Control (FfCtl) ==
  FfCtl_FfCtlRatio_C : Inport
  FfCtl_vVehSpd : Inport  Port=2
  FfCtl_crPrvwCrvt : Inport  Port=3
  FfCtl_lWhlBase_SY : Inport  Port=4
  FfCtl_rTraRatio_C : Inport  Port=5
  Add : Sum  OutDataTypeStr=single
  Constant1 : Constant  OutDataTypeStr=single
  Divide : Product  Inputs=*/  OutDataTypeStr=single
  Divide1 : Product  Inputs=*/  OutDataTypeStr=single
  Gain2 : Gain  Gain=-1  OutDataTypeStr=single
  Lookup Table2 : Lookup_n-D  NumberOfTableDimensions=1  BreakpointsForDimension1=[11.7,18.83,26.98,31.98,51.04,79,86.08,90.59]  BeginIndexSearchUsingPreviousIndexResult=on  Table=[0.012141,0.005179,0.00298,0.002547,0.001715,0.001283,0.001021,0.000982]  DiagnosticForOutOfRangeInput=Warning  RemoveProtectionInput=on  InternalRulePriority=Speed  OutDataTypeStr=single  InputSameDT=on
  Math Function : Math  Operator=magnitude^2  OutDataTypeStr=single  SaturateOnIntegerOverflow=on
  Product : Product  OutDataTypeStr=single
  Product1 : Product  OutDataTypeStr=single
  Product2 : Product  OutDataTypeStr=single
  Product3 : Product  Inputs=3  OutDataTypeStr=single
  Saturation1 : Saturate  UpperLimit=0.01  LowerLimit=0
  kph to mps : Gain  Gain=1/3.6  OutDataTypeStr=single
  rad to deg : Gain  Gain=180/pi  OutDataTypeStr=single
  FfCtl_phiFfSWA : Outport
  wires:
  Gain2/1 -> FfCtl_phiFfSWA/1
  kph to mps/1 -> Divide/1, Math Function/1, Product/1
  rad to deg/1 -> Product1/1
  Product1/1 -> Product3/2
  Divide1/1 -> Product1/2
  Divide/1 -> Divide1/2
  FfCtl_lWhlBase_SY/1 -> Divide/2
  Add/1 -> Divide1/1
  Constant1/1 -> Add/2
  Product2/1 -> Add/1
  Math Function/1 -> Product2/1
  Product/1 -> rad to deg/1
  FfCtl_crPrvwCrvt/1 -> Product/2
  FfCtl_vVehSpd/1 -> Lookup Table2/1, kph to mps/1
  Product3/1 -> Gain2/1
  FfCtl_rTraRatio_C/1 -> Product3/3
  FfCtl_FfCtlRatio_C/1 -> Product3/1
  Lookup Table2/1 -> Saturation1/1
  Saturation1/1 -> Product2/2  "FfCtl_facmUSG_C"

== system LKAS_AutoSave_20200911_1102/LKAS/LL/LLOn/LKA/Plan To LaneFollowing (PTLF)/InsideJudge1/If Action Subsystem ==
  T1 : Inport
  Plan : Inport  Port=2
  HdAgLft : Inport  Port=3
  Time : Inport  Port=4
  Action Port : ActionPort  InitializeStates=reset  ActionType=then
  Add : Sum
  Cast To Single : DataTypeConversion  OutDataTypeStr=uint8
  Compare To Constant : simulink/Logic and Bit Operations/Compare To Constant  relop=>=  const=0  OutDataTypeStr=boolean
  Detect Decrease : simulink/Logic and Bit Operations/Detect Decrease  vinit=0.0  OutDataTypeStr=boolean
  If Action Subsystem : Subsystem  TreatAsAtomicUnit=on
  If Action Subsystem2 : Subsystem  TreatAsAtomicUnit=on
  Logical Operator : Logic  AllPortsSameDT=off  OutDataTypeStr=boolean
  Memory : Memory  InheritSampleTime=on
  Relational Operator : RelationalOperator  OutDataTypeStr=boolean  RndMeth=Simplest
  Saturation : Saturate  UpperLimit=5  LowerLimit=0
  Switch : Switch  Criteria=u2 > Threshold
  Switch1 : Switch  Criteria=u2 > Threshold
  T1_1 : Outport
  Plan_1 : Outport  Port=2
  wires:
  HdAgLft/1 -> Compare To Constant/1
  Compare To Constant/1 -> Detect Decrease/1
  Time/1 -> If Action Subsystem/1(T1), Relational Operator/2
  Plan/1 -> If Action Subsystem2/2(Plan), If Action Subsystem/2(Plan)
  T1/1 -> If Action Subsystem2/1(T1), Relational Operator/1
  Detect Decrease/1 -> Logical Operator/1
  Relational Operator/1 -> Logical Operator/2
  Add/1 -> Saturation/1
  Memory/1 -> Add/2
  Logical Operator/1 -> Cast To Single/1
  Cast To Single/1 -> Add/1
  Saturation/1 -> Switch1/2, Switch/2, If Action Subsystem/Enable, Memory/1
  If Action Subsystem/1(T1_1) -> Switch/1
  If Action Subsystem/2(Plan_1) -> Switch1/1
  If Action Subsystem2/1(T1_1) -> Switch/3
  If Action Subsystem2/2(Plan_1) -> Switch1/3
  Switch/1 -> T1_1/1
  Switch1/1 -> Plan_1/1

== system LKAS_AutoSave_20200911_1102/LKAS/LL/LLOn/LKA/Plan To LaneFollowing (PTLF)/InsideJudge1/If Action Subsystem1 ==
  T1 : Inport
  Plan : Inport  Port=2
  HdAgRgt : Inport  Port=3
  Time : Inport  Port=4
  Action Port : ActionPort  InitializeStates=reset  ActionType=elseif
  Add : Sum
  Cast To Single : DataTypeConversion  OutDataTypeStr=uint8
  Compare To Constant : simulink/Logic and Bit Operations/Compare To Constant  relop=<=  const=0  OutDataTypeStr=boolean
  Detect Decrease : simulink/Logic and Bit Operations/Detect Decrease  vinit=0.0  OutDataTypeStr=boolean
  If Action Subsystem : Subsystem  TreatAsAtomicUnit=on
  If Action Subsystem2 : Subsystem  TreatAsAtomicUnit=on
  Logical Operator : Logic  AllPortsSameDT=off  OutDataTypeStr=boolean
  Memory : Memory  InheritSampleTime=on
  Relational Operator : RelationalOperator  OutDataTypeStr=boolean  RndMeth=Simplest
  Saturation : Saturate  UpperLimit=5  LowerLimit=0
  Switch : Switch  Criteria=u2 > Threshold
  Switch1 : Switch  Criteria=u2 > Threshold
  T1_1 : Outport
  Plan_1 : Outport  Port=2
  wires:
  Relational Operator/1 -> Logical Operator/2
  Detect Decrease/1 -> Logical Operator/1
  Compare To Constant/1 -> Detect Decrease/1
  HdAgRgt/1 -> Compare To Constant/1
  Time/1 -> Relational Operator/2, If Action Subsystem/1(T1)
  Add/1 -> Saturation/1
  T1/1 -> If Action Subsystem2/1(T1), Relational Operator/1
  Memory/1 -> Add/2
  Logical Operator/1 -> Cast To Single/1
  Cast To Single/1 -> Add/1
  Saturation/1 -> Memory/1, Switch1/2, Switch/2, If Action Subsystem/Enable
  If Action Subsystem2/1(T1_1) -> Switch/3
  If Action Subsystem/2(Plan_1) -> Switch1/1
  Switch/1 -> T1_1/1
  Switch1/1 -> Plan_1/1
  If Action Subsystem2/2(Plan_1) -> Switch1/3
  If Action Subsystem/1(T1_1) -> Switch/1
  Plan/1 -> If Action Subsystem/2(Plan), If Action Subsystem2/2(Plan)

== system LKAS_AutoSave_20200911_1102/LKAS/LL/LLOn/LKA/Plan To LaneFollowing (PTLF)/InsideJudge1/If Action Subsystem2 ==
  T1 : Inport
  Plan : Inport  Port=2
  Action Port : ActionPort  InitializeStates=reset  ActionType=else
  T1_1 : Outport
  Plan_1 : Outport  Port=2
  wires:
  T1/1 -> T1_1/1
  Plan/1 -> Plan_1/1

== system LKAS_AutoSave_20200911_1102/LKAS/LL/LLOn/LKA Input Processing (LKAInP)/Predicted Deviation Calculation (PrDvt)/Lane Information Selection (LaneInfoSel)/If Action Subsystem1 ==
  In1 : Inport
  Action Port : ActionPort  InitializeStates=reset  ActionType=elseif
  Out1 : Outport
  wires:
  In1/1 -> Out1/1

== system LKAS_AutoSave_20200911_1102/LKAS/LL/LLOn/LKA Input Processing (LKAInP)/Predicted Deviation Calculation (PrDvt)/Lane Information Selection (LaneInfoSel)/If Action Subsystem2 ==
  In1 : Inport
  Action Port : ActionPort  InitializeStates=reset  ActionType=then
  Out1 : Outport
  wires:
  In1/1 -> Out1/1

== system LKAS_AutoSave_20200911_1102/LKAS/LL/LLOn/LKA Input Processing (LKAInP)/Predicted Deviation Calculation (PrDvt)/Lane Information Selection (LaneInfoSel)/If Action Subsystem3 ==
  In1 : Inport
  In2 : Inport  Port=2
  Action Port : ActionPort  InitializeStates=reset  ActionType=else
  Add : Sum
  Gain : Gain  Gain=0.5
  Out1 : Outport
  wires:
  Gain/1 -> Out1/1
  In1/1 -> Add/1
  In2/1 -> Add/2
  Add/1 -> Gain/1

== system LKAS_AutoSave_20200911_1102/LKAS/LL/LLOn/LKA Input Processing (LKAInP)/Predicted Deviation Calculation (PrDvt)/Lane Information Selection (LaneInfoSel)1/If Action Subsystem1 ==
  In1 : Inport
  Action Port : ActionPort  InitializeStates=reset  ActionType=elseif
  Out1 : Outport
  wires:
  In1/1 -> Out1/1

== system LKAS_AutoSave_20200911_1102/LKAS/LL/LLOn/LKA Input Processing (LKAInP)/Predicted Deviation Calculation (PrDvt)/Lane Information Selection (LaneInfoSel)1/If Action Subsystem2 ==
  In1 : Inport
  Action Port : ActionPort  InitializeStates=reset  ActionType=then
  Out1 : Outport
  wires:
  In1/1 -> Out1/1

== system LKAS_AutoSave_20200911_1102/LKAS/LL/LLOn/LKA Input Processing (LKAInP)/Predicted Deviation Calculation (PrDvt)/Lane Information Selection (LaneInfoSel)1/If Action Subsystem3 ==
  In1 : Inport
  In2 : Inport  Port=2
  Action Port : ActionPort  InitializeStates=reset  ActionType=else
  Min : MinMax  Inputs=2
  Out1 : Outport
  wires:
  In2/1 -> Min/2
  In1/1 -> Min/1
  Min/1 -> Out1/1

== system LKAS_AutoSave_20200911_1102/LKAS/LL/LLOn/LKA Input Processing (LKAInP)/Predicted Heading Angle Calculation (PrHdAg)/Lane Information Selection (LaneInfoSel)/If Action Subsystem1 ==
  In1 : Inport
  Action Port : ActionPort  InitializeStates=reset  ActionType=elseif
  Out1 : Outport
  wires:
  In1/1 -> Out1/1

== system LKAS_AutoSave_20200911_1102/LKAS/LL/LLOn/LKA Input Processing (LKAInP)/Predicted Heading Angle Calculation (PrHdAg)/Lane Information Selection (LaneInfoSel)/If Action Subsystem2 ==
  In1 : Inport
  Action Port : ActionPort  InitializeStates=reset  ActionType=then
  Out1 : Outport
  wires:
  In1/1 -> Out1/1

== system LKAS_AutoSave_20200911_1102/LKAS/LL/LLOn/LKA Input Processing (LKAInP)/Predicted Heading Angle Calculation (PrHdAg)/Lane Information Selection (LaneInfoSel)/If Action Subsystem3 ==
  In1 : Inport
  In2 : Inport  Port=2
  Action Port : ActionPort  InitializeStates=reset  ActionType=else
  Add : Sum
  Gain : Gain  Gain=0.5
  Out1 : Outport
  wires:
  Gain/1 -> Out1/1
  Add/1 -> Gain/1
  In1/1 -> Add/1
  In2/1 -> Add/2

== system LKAS_AutoSave_20200911_1102/LKAS/LL/LLOn/LKA Input Processing (LKAInP)/Predicted Heading Angle Calculation (PrHdAg)/Lane Information Selection (LaneInfoSel)1/If Action Subsystem1 ==
  In1 : Inport
  Action Port : ActionPort  InitializeStates=reset  ActionType=elseif
  Out1 : Outport
  wires:
  In1/1 -> Out1/1

== system LKAS_AutoSave_20200911_1102/LKAS/LL/LLOn/LKA Input Processing (LKAInP)/Predicted Heading Angle Calculation (PrHdAg)/Lane Information Selection (LaneInfoSel)1/If Action Subsystem2 ==
  In1 : Inport
  Action Port : ActionPort  InitializeStates=reset  ActionType=then
  Out1 : Outport
  wires:
  In1/1 -> Out1/1

== system LKAS_AutoSave_20200911_1102/LKAS/LL/LLOn/LKA Input Processing (LKAInP)/Predicted Heading Angle Calculation (PrHdAg)/Lane Information Selection (LaneInfoSel)1/If Action Subsystem3 ==
  In1 : Inport
  In2 : Inport  Port=2
  Action Port : ActionPort  InitializeStates=reset  ActionType=else
  Add : Sum
  Gain : Gain  Gain=0.5
  Out1 : Outport
  wires:
  In2/1 -> Add/2
  In1/1 -> Add/1
  Add/1 -> Gain/1
  Gain/1 -> Out1/1

== system LKAS_AutoSave_20200911_1102/LKAS/LL/LLOn/LKA Input Processing (LKAInP)/Predicted Heading Angle Calculation (PrHdAg)/Perdicted Heading Angle Compensation (PrdcHdAgComp)/Yaw Rate Stable Gain (YRSG) ==
  YRSG_vVehSpd : Inport
  Add : Sum  OutDataTypeStr=single
  Bus Selector : BusSelector  OutputSignals=LKA_WhlBaseL_C
  Divide2 : Product  Inputs=*/  OutDataTypeStr=single
  Divide3 : Product  Inputs=*/  OutDataTypeStr=single
  Lookup Table2 : Lookup_n-D  NumberOfTableDimensions=1  BreakpointsForDimension1=[11.7,18.83,26.98,31.98,51.04,79,86.08,90.59]  BeginIndexSearchUsingPreviousIndexResult=on  Table=[0.012141,0.005179,0.00298,0.002547,0.001715,0.001283,0.001021,0.000982]  DiagnosticForOutOfRangeInput=Warning  RemoveProtectionInput=on  InternalRulePriority=Speed  OutDataTypeStr=single  InputSameDT=on
  Product1 : Product  Inputs=3  OutDataTypeStr=single
  Saturation1 : Saturate  UpperLimit=0.012141  LowerLimit=0.000982
  "constant " : Constant  OutDataTypeStr=single
  kph To mps : Gain  Gain=1/3.6  OutDataTypeStr=single
  YRSG_dphiYRSG : Outport
  wires:
  kph To mps/1 -> Divide2/1, Product1/1, Product1/2
  Saturation1/1 -> Product1/3
  Lookup Table2/1 -> Saturation1/1
  Divide3/1 -> YRSG_dphiYRSG/1
  Add/1 -> Divide3/2
  "constant "/1 -> Add/2
  Product1/1 -> Add/1
  Divide2/1 -> Divide3/1
  Bus Selector/1 -> Divide2/2  "<LKA_WhlBaseL_C>"
  YRSG_vVehSpd/1 -> Lookup Table2/1, kph To mps/1
  [LLClb_bsConstantClb] -> Bus Selector/1

== system LKAS_AutoSave_20200911_1102/LKAS/LL/LLOn/LKA Input Processing (LKAInP)/Previewed Curvature (PrCrvt)/Lane Information Selection (LaneInfoSel)/If Action Subsystem1 ==
  In1 : Inport
  Action Port : ActionPort  InitializeStates=reset  ActionType=elseif
  Out1 : Outport
  wires:
  In1/1 -> Out1/1

== system LKAS_AutoSave_20200911_1102/LKAS/LL/LLOn/LKA Input Processing (LKAInP)/Previewed Curvature (PrCrvt)/Lane Information Selection (LaneInfoSel)/If Action Subsystem2 ==
  In1 : Inport
  Action Port : ActionPort  InitializeStates=reset  ActionType=then
  Out1 : Outport
  wires:
  In1/1 -> Out1/1

== system LKAS_AutoSave_20200911_1102/LKAS/LL/LLOn/LKA Input Processing (LKAInP)/Previewed Curvature (PrCrvt)/Lane Information Selection (LaneInfoSel)/If Action Subsystem3 ==
  In1 : Inport
  In2 : Inport  Port=2
  Action Port : ActionPort  InitializeStates=reset  ActionType=else
  Add : Sum
  Gain : Gain  Gain=0.5
  Out1 : Outport
  wires:
  Gain/1 -> Out1/1
  In1/1 -> Add/1
  In2/1 -> Add/2
  Add/1 -> Gain/1
